simulink model "problem6cascademodel"  (R2020b)
settings: Solver=VariableStepAuto  StartTime=0.0  StopTime=10.0  RelTol=1e-3
settings Model: Creator=admin  LastModifiedBy=admin

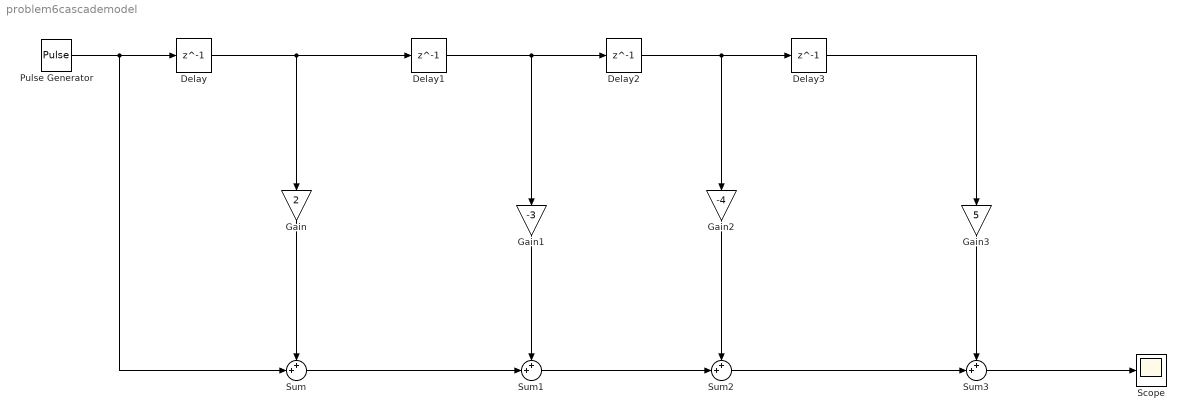
== system problem6cascademodel ==
  Delay{,1..3} (4 alike) : Delay  DelayLength=1  InitialCondition=0
  Gain : Gain  Gain=2
  Gain1 : Gain  Gain=-3
  Gain2 : Gain  Gain=-4
  Gain3 : Gain  Gain=5
  Pulse Generator : DiscretePulseGenerator  PulseType=Time based  Period=10  PulseWidth=5
  Scope : Scope
  Sum{,1..3} (4 alike) : Sum  Inputs=++|
  wires:
  Delay3/1 -> Gain3/1
  Gain3/1 -> Sum3/1
  Sum3/1 -> Scope/1
  Sum2/1 -> Sum3/2
  Delay1/1 -> Delay2/1, Gain1/1
  Delay/1 -> Delay1/1, Gain/1
  Pulse Generator/1 -> Sum/2, Delay/1
  Sum1/1 -> Sum2/2
  Sum/1 -> Sum1/2
  Gain1/1 -> Sum1/1
  Gain/1 -> Sum/1
  Gain2/1 -> Sum2/1
  Delay2/1 -> Gain2/1, Delay3/1
